simulink model "DSB_FC"  (R2023a)
settings: Solver=VariableStepAuto  StartTime=0.0  StopTime=1  RelTol=1e-3
libraries: dspfdesign x1
settings Model: Creator=dung  LastModifiedBy=dung

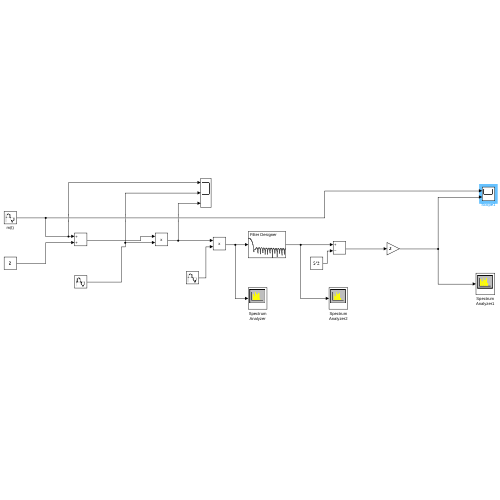
[thumbnail: Simulink's stored preview of the top-level diagram]
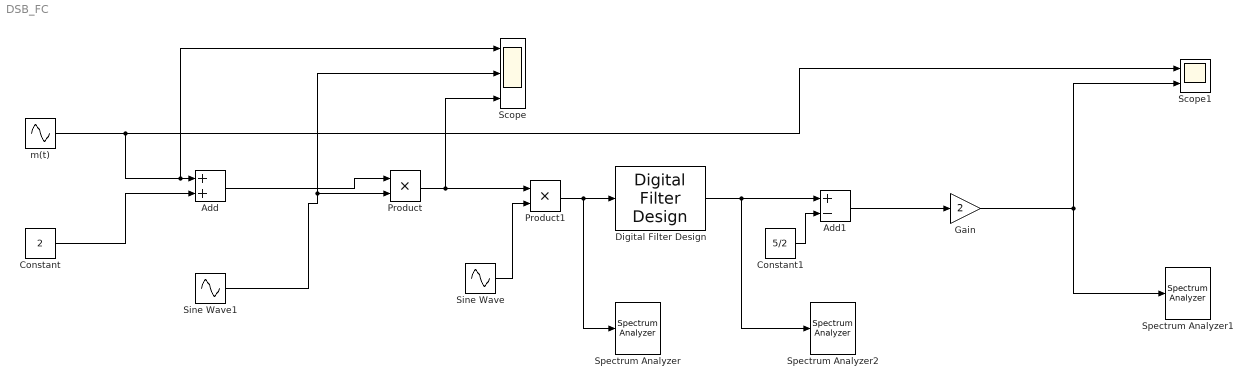
== system DSB_FC ==
  Add : Sum
  Add1 : Sum  Inputs=+-
  Constant : Constant  Value=2
  Constant1 : Constant  Value=5/2
  Digital Filter Design : dspfdesign/Digital Filter Design  mwdsp_browser_bugfix_var=off
  Gain : Gain  Gain=2
  Product : Product
  Product1 : Product
  Scope : Scope  NumInputPorts=3
  Scope1 : Scope  NumInputPorts=2
  Sine Wave : Sin  Frequency=2*pi*5000  SampleTime=1/50000
  Sine Wave1 : Sin  Frequency=2*pi*5000  SampleTime=1/50000
  Spectrum Analyzer : SpectrumAnalyzer  WindowPosition=[1.000000,12.000000,1397.000000,752.000000,]  ScopeFrameLocation=window  Span=49999.99999999999  StartFrequency=-24999.999999999996  StopFrequency=24999.999999999996  YLimits=[-132.5639802,48.03143359]  ColorLimits=[-20 80]  DefaultConfigurationName=spbscopes.SpectrumAnalyzerBlockCfg  IsFrequencyInputMode=0  FrequencyVectorPort=0  FrequencyVectorFromPort=0  FrequencyInputRBWPort=0  FrequencyInputRBWFromPort=0
  Spectrum Analyzer1 : SpectrumAnalyzer  WindowPosition=[560.000000,150.000000,1078.000000,640.000000,]  ScopeFrameLocation=window  YLimits=[-62.29188714,50.82597248]  ColorLimits=[-20 80]  DefaultConfigurationName=spbscopes.SpectrumAnalyzerBlockCfg  IsFrequencyInputMode=0  FrequencyVectorPort=0  FrequencyVectorFromPort=0  FrequencyInputRBWPort=0  FrequencyInputRBWFromPort=0
  Spectrum Analyzer2 : SpectrumAnalyzer  WindowPosition=[325.000000,239.000000,921.000000,535.000000,]  ScopeFrameLocation=window  YLimits=[-194.02922194,54.86080904]  ColorLimits=[-20 80]  DefaultConfigurationName=spbscopes.SpectrumAnalyzerBlockCfg  IsFrequencyInputMode=0  FrequencyVectorPort=0  FrequencyVectorFromPort=0  FrequencyInputRBWPort=0  FrequencyInputRBWFromPort=0
  m(t) : Sin  Frequency=2*pi*200  SampleTime=1/50000
  wires:
  m(t)/1 -> Scope1/1, Scope/1, Add/1
  Constant/1 -> Add/2
  Add/1 -> Product/1
  Sine Wave1/1 -> Scope/2, Product/2
  Product/1 -> Scope/3, Product1/1
  Add1/1 -> Gain/1
  Digital Filter Design/1 -> Add1/1, Spectrum Analyzer2/1
  Constant1/1 -> Add1/2
  Gain/1 -> Scope1/2, Spectrum Analyzer1/1
  Sine Wave/1 -> Product1/2
  Product1/1 -> Spectrum Analyzer/1, Digital Filter Design/1
